simulink model "sampling"  (R2019a)
settings: Solver=VariableStepAuto  StartTime=0.0  StopTime=10.0  RelTol=1e-3
libraries: dspsigops x1
settings Model: Creator=susiejojo  LastModifiedBy=susiejojo

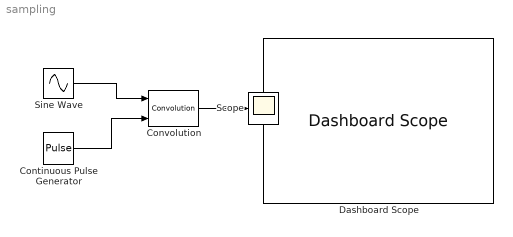
== system sampling ==
  Continuous Pulse Generator : DiscretePulseGenerator  PulseType=Time based  Period=0.10  PulseWidth=50
  Convolution : dspsigops/Convolution  domain=Time  roundingMode=Floor  overflowMode=off  outputDataTypeStr=Inherit: Same as accumulator  outputMin=[]  outputMax=[]  outputLastDataTypeStr=Inherit: Same as accumulator
      settings: SourceProductName=DSP System Toolbox  SourceProductBaseCode=DS
  Dashboard Scope : DashboardScope  LegendPosition=Right
  Scope : Scope
  Sine Wave : Sin  Frequency=2  SampleTime=0
  wires:
  Continuous Pulse Generator/1 -> Convolution/2
  Sine Wave/1 -> Convolution/1
  Convolution/1 -> Scope/1
